simulink model "PID2"  (R2017b)
settings: Solver=ode5  StartTime=0.0  StopTime=10.0  FixedStep=0.0001  RelTol=1e-3
values from neighbouring files (symbols this model uses):
  aa = 420    [GA_fitfun_EXPID2.m]
  bb = 35    [GA_fitfun_EXPID2.m]
  cc = 200    [GA_fitfun_EXPID2.m]
  Kd = minium_Kp_Ki_Kd(3)    [EXPID1.m]    (also in GA_fitfun_EXPID1.m = chro(3); GA_fitfun_EXPID2.m = chro(3))
  Ki = minium_Kp_Ki_Kd(2)    [EXPID1.m]    (also in GA_fitfun_EXPID1.m = chro(2); GA_fitfun_EXPID2.m = chro(2))
  Kp = minium_Kp_Ki_Kd(1)    [EXPID1.m]    (also in GA_fitfun_EXPID1.m = chro(1); GA_fitfun_EXPID2.m = chro(1))
settings Model: Creator=Yenchun  LastModifiedBy=liyenjun
settings CodeAppCC: StateflowObjectComments=on

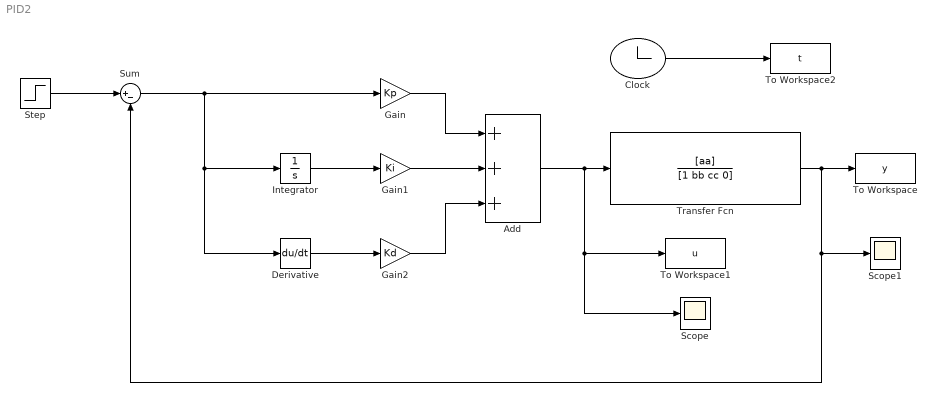
== system PID2 ==
  Add : Sum  Inputs=+++
  Clock : Clock
  Derivative : Derivative
  Gain : Gain  Gain=Kp
  Gain1 : Gain  Gain=Ki
  Gain2 : Gain  Gain=Kd
  Integrator : Integrator
  Scope : Scope
  Scope1 : Scope
  Step : Step  Before=1  SampleTime=0
  Sum : Sum  Inputs=|+-
  To Workspace : ToWorkspace  VariableName=y  SampleTime=-1
      settings: Save2DSignal=2-D array (concatenate along first dimension)
  To Workspace1 : ToWorkspace  VariableName=u  SampleTime=-1
      settings: Save2DSignal=2-D array (concatenate along first dimension)
  To Workspace2 : ToWorkspace  VariableName=t  SampleTime=-1
      settings: Save2DSignal=2-D array (concatenate along first dimension)
  Transfer Fcn : TransferFcn  Numerator=[aa]  Denominator=[1 bb cc 0]
  wires:
  Step/1 -> Sum/1
  Integrator/1 -> Gain1/1
  Derivative/1 -> Gain2/1
  Sum/1 -> Derivative/1, Integrator/1, Gain/1
  Gain/1 -> Add/1
  Gain1/1 -> Add/2
  Gain2/1 -> Add/3
  Add/1 -> Scope/1, To Workspace1/1, Transfer Fcn/1
  Transfer Fcn/1 -> Sum/2, Scope1/1, To Workspace/1
  Clock/1 -> To Workspace2/1
